simulink model "reg"  (R2024b)
settings: Solver=VariableStepAuto  StartTime=tspan(1)  StopTime=tspan(2)  RelTol=1e-3
values from neighbouring files (symbols this model uses):
  den = [1 1 0.2]    [main.m]
  desr = [35 40]    [main.m]
  desr_val = 0.5    [main.m]
  num = 0.1    [main.m]
  Reg = ButtwPICoef    [main.m]
  step_t = 5    [main.m]
  u_des = 1    [main.m]
settings Model: Creator=markminerov  LastModifiedBy=markminerov

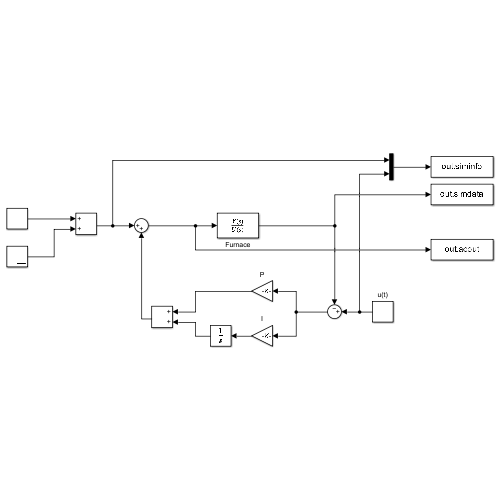
[thumbnail: Simulink's stored preview of the top-level diagram]
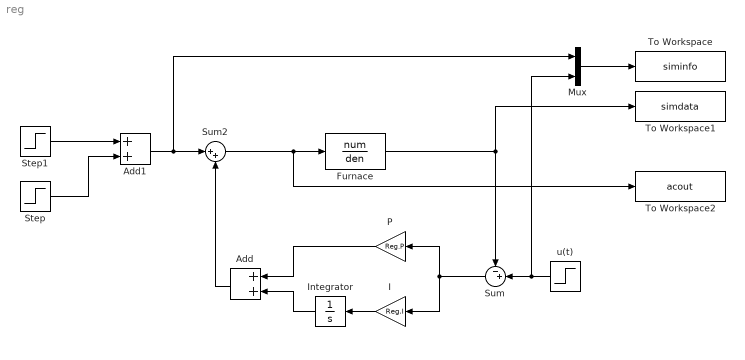
== system reg ==
  Add : Sum
  Add1 : Sum
  Furnace : TransferFcn  Numerator=num  Denominator=den
  I : Gain  Gain=Reg.I
  Integrator : Integrator
  Mux : Mux  Inputs=2
  P : Gain  Gain=Reg.P
  Step : Step  Time=desr(1)  After=-desr_val  SampleTime=0
  Step1 : Step  Time=desr(2)  After=desr_val  SampleTime=0
  Sum : Sum  Inputs=-+|
  Sum2 : Sum  Inputs=|++
  To Workspace : ToWorkspace  VariableName=siminfo  SaveFormat=Timeseries  SampleTime=-1
  To Workspace1 : ToWorkspace  VariableName=simdata  SaveFormat=Timeseries  SampleTime=-1
  To Workspace2 : ToWorkspace  VariableName=acout  SaveFormat=Timeseries  SampleTime=-1
  u(t) : Step  Time=step_t  After=u_des  SampleTime=0
  wires:
  Furnace/1 -> Sum/1, To Workspace1/1
  Sum/1 -> I/1, P/1
  P/1 -> Add/1
  Integrator/1 -> Add/2
  I/1 -> Integrator/1
  u(t)/1 -> Mux/2, Sum/2
  Step1/1 -> Add1/1
  Step/1 -> Add1/2
  Add/1 -> Sum2/2
  Add1/1 -> Mux/1, Sum2/1
  Sum2/1 -> To Workspace2/1, Furnace/1
  Mux/1 -> To Workspace/1
